simulink model "LQ_simulation"  (R2018a)
settings: Solver=ode45  StartTime=0.0  StopTime=50  RelTol=1e-3  EnableMultiTasking=on
values from neighbouring files (symbols this model uses):
  h = 0.001    [LQ_main.m]
  K = K_lqi(1:4)    [LQ_main.m]
  Ki = K_lqi(5:6)    [LQ_main.m]
  R_kal = cov(err)    [LQ_main.m]
undefined symbols (not defined in the file or in its folder): DiscIntNeverNeededParam, Discrete, get, hot, Time
libraries: simulink x2, ctrlSharedLib x1, dspmtrx3 x1, dspsnks4 x1
settings Model: Creator=rbabuska  LastModifiedBy=sstroobants
settings DataIOCC: LimitDataPoints=on  SaveFormat=Array  SignalLoggingName=sigsOut
settings OptimizationCC: BooleanDataType=off  ExpressionDepthLimit=2147483647  InitFltsAndDblsToZero=on  LifeSpan=inf
settings DebuggingCC: SaveWithParameterizedLinksMsg=none  SignalResolutionControl=TryResolveAllWithWarning  MultiTaskDSMMsg=warning  MultiTaskCondExecSysMsg=none  AllowSymbolicDim=off  StateNameClashWarn=warning  SFUnexpectedBacktrackingDiag=warning  SFNoUnconditionalDefaultTransitionDiag=warning  SFExecutionAtInitializationDiag=none
settings HardwareCC: ProdBitPerPointer=32  ProdBitPerSizeT=32  ProdBitPerPtrDiffT=32  ProdLargestAtomicFloat=None  ProdIntDivRoundTo=Undefined  ProdEndianess=Unspecified  ProdWordSize=32  ProdHWDeviceType=32-bit Generic  TargetUnknown=on
settings ModelReferenceCC: PropagateSignalLabelsOutOfModel=off
settings CodeAppCC: StateflowObjectComments=on
settings GRTTargetCC: TargetFcnLib=ansi_tfl_tmw.mat  TargetLangStandard=C89/C90 (ANSI)  GeneratePreprocessorConditionals=Disable all  CombineOutputUpdateFcns=off  GRTInterface=on
settings ConfigComp: CovMetricSettings=dw  CovHtmlReporting=on  CovSaveCumulativeToWorkspaceVar=on  CovSaveSingleToWorkspaceVar=on  CovExternalEMLEnable=off

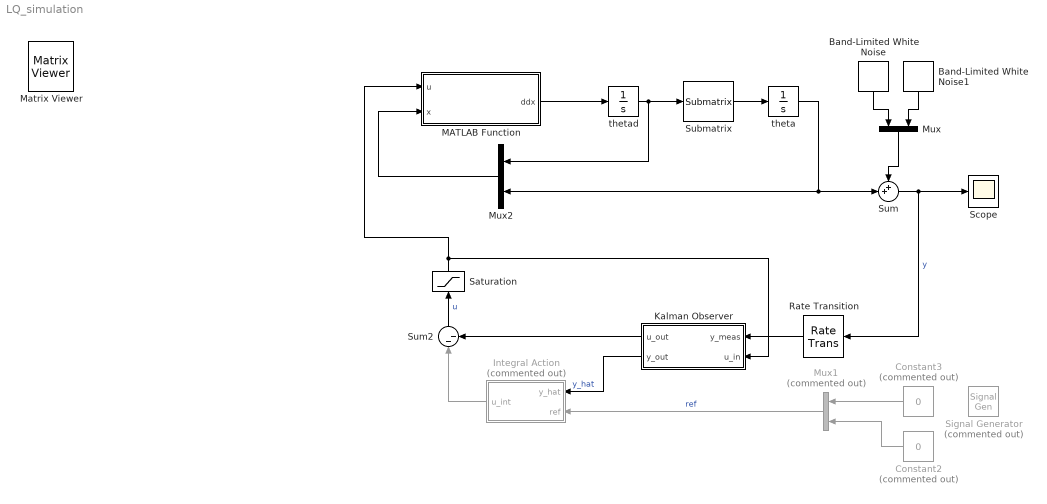
== system LQ_simulation ==
  Band-Limited White Noise : simulink/Sources/Band-Limited White Noise  Cov=R_kal(1,1)*h  Ts=h  seed=[23341]
  Band-Limited White Noise1 : simulink/Sources/Band-Limited White Noise  Cov=R_kal(2,2)*h  Ts=h  seed=[23341]
  Constant2 : Constant  Commented=on  Value=0
  Constant3 : Constant  Commented=on  Value=0
  Integral Action : Subsystem  Commented=on
  Kalman Observer : Subsystem
  MATLAB Function : MATLAB Function  TreatAsAtomicUnit=on  SystemSampleTime=h
  Mux : Mux  Inputs=2
  Mux1 : Mux  Commented=on  Inputs=2
  Mux2 : Mux  Inputs=2
  Rate Transition : RateTransition  OutPortSampleTime=h
  Saturation : Saturate  UpperLimit=1  LowerLimit=-1
  Scope : Scope
  Signal Generator : SignalGenerator  Commented=on  WaveForm=square  Amplitude=0.3  Frequency=0.2  Units=rad/sec
  Submatrix : dspmtrx3/Submatrix  RowSpan=Range of rows  RowStartMode=First  RowStartIndex=1  RowEndMode=Index  RowEndIndex=2  ColSpan=Range of columns  ColStartMode=First  ColStartIndex=1  ColEndMode=Last  ColEndIndex=1
  Sum : Sum  Inputs=++|
  Sum2 : Sum  Inputs=|--
  theta : Integrator  InitialCondition=[0;0]
  thetad : Integrator  InitialCondition=[0 0 0]
  Matrix Viewer : dspsnks4/Matrix Viewer  IOType=viewer  ImageParams=off  CMapStr=hot(256)  AxisColorbar=on  AxisParams=off  AxisOrigin=Upper left corner  AxisTickMode=Auto  XTickRange=[0 1]  YTickRange=[0 1]  XLabel=X-axis  YLabel=Y-axis  ZLabel=Z-axis  FigPos=get(0,'defaultfigureposition')  AxisZoom=off
      settings: SourceProductName=DSP System Toolbox  SourceProductBaseCode=DS  YMin=-1.0  YMax=1.0
  wires:
  Sum2/1 -> Saturation/1  "u"
  Saturation/1 -> MATLAB Function/1(u), Kalman Observer/2(u_in)
  Sum/1 -> Scope/1, Rate Transition/1  "y"
  Kalman Observer/1(u_out) -> Sum2/2
  Mux/1 -> Sum/1
  Band-Limited White Noise/1 -> Mux/1
  Band-Limited White Noise1/1 -> Mux/2
  Kalman Observer/2(y_out) -> Integral Action/1(y_hat)  "y_hat"
  Integral Action/1(u_int) -> Sum2/1
  Mux1/1 -> Integral Action/2(ref)  "ref"
  Constant2/1 -> Mux1/2
  Constant3/1 -> Mux1/1
  Mux2/1 -> MATLAB Function/2(x)
  Submatrix/1 -> theta/1
  thetad/1 -> Submatrix/1, Mux2/1
  MATLAB Function/1(ddx) -> thetad/1
  theta/1 -> Sum/2, Mux2/2
  Rate Transition/1 -> Kalman Observer/1(y_meas)

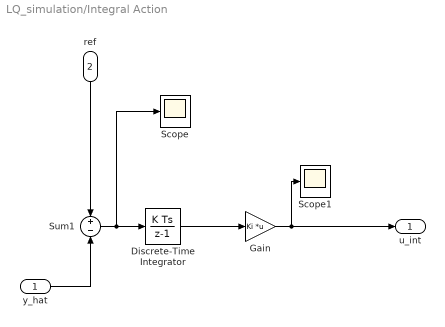
== system LQ_simulation/Integral Action ==
  y_hat : Inport
  ref : Inport  Port=2
  Discrete-Time Integrator : DiscreteIntegrator  gainval=1.5  SampleTime=h  ICPrevOutput=DiscIntNeverNeededParam  ICPrevScaledInput=DiscIntNeverNeededParam
  Gain : Gain  Gain=Ki  Multiplication=Matrix(K*u)
  Scope : Scope
  Scope1 : Scope
  Sum1 : Sum  Inputs=+-
  u_int : Outport
  wires:
  ref/1 -> Sum1/1
  y_hat/1 -> Sum1/2
  Sum1/1 -> Scope/1, Discrete-Time Integrator/1
  Discrete-Time Integrator/1 -> Gain/1
  Gain/1 -> Scope1/1, u_int/1

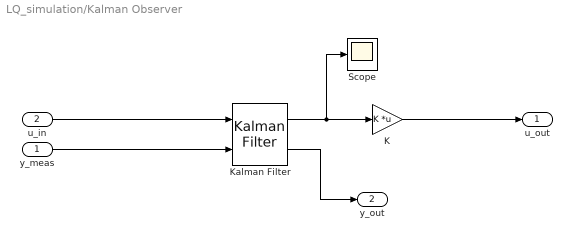
== system LQ_simulation/Kalman Observer ==
  y_meas : Inport  PortDimensions=2
  u_in : Inport  Port=2  PortDimensions=1  SampleTime=h
  K : Gain  Gain=K  Multiplication=Matrix(K*u)
  Kalman Filter : ctrlSharedLib/Kalman Filter  TimeDomain=Discrete-Time  UseCurrentEstimator=on  ModelSource=LTI State-Space Variable  ModelSourceVariable=sysd  A=0.95  B=1  C=1  D=0  NumberOfStates=1  NumberOfInputs=1  NumberOfOutputs=1  InitialEstimateSource=Dialog  X0=0  P0=10  UseK=off  UseGH=off  NumberOfProcessNoiseInputs=1  G=1  TimeInvariantG=on  H=0  TimeInvariantH=on  Q=10^(-7)*eye(4)  TimeInvariantQ=on  R=R_kal  TimeInvariantR=on  N=0  TimeInvariantN=on  AddInputPort=on  AddEnablePort=off  OutputEstimatedY=on  OutputP=off  Ts=-1
      settings: SourceProductBaseCode=CT
  Scope : Scope
  u_out : Outport
  y_out : Outport  Port=2
  wires:
  K/1 -> u_out/1
  u_in/1 -> Kalman Filter/1
  y_meas/1 -> Kalman Filter/2
  Kalman Filter/1 -> Scope/1, K/1
  Kalman Filter/2 -> y_out/1

== matlab function LQ_simulation/MATLAB Function ==
  data: u input; x input; ddx output
function ddx = nonlinsim(u,x)
theta1  = x(4);
theta2  = x(5);
theta1d = x(1);
theta2d = x(2);
ii      = x(3);
par =     [0.107001615392530   0.165343973632010   0.040783104942133   0.046364080778153   0.000051655820835   0.048856187724916   0.049137116812930   1.636038234993470   0.000031810472615   1.827977549139487   0.000008590269497   0.006045619229031   3.032790298604742   0.098524631245120   1.049678153165582];

%Define parameters
L1 = par(1);m1 = par(2);m2 = par(3); I1 = par(4); I2 = par(5);
c1 = par(6); c2 = par(7); 
b1 = par(8); b2 = par(9);  Bc1 = par(10); Bc2 = par(11);
 L = par(12); Kt = par(13); R = par(14); Kv = par(15);
g = 9.81;
M = -7;
%Input
Tau = u;%interp1(u.Time,u.Data,t);
ddx = zeros(3,1);
% dx(1) = x(3);
% dx(2) = x(4);
ddx(1) = (3*I2*Kt*ii - 2*Bc2*I2*atan(500*theta1d - 500*theta2d) - 2*Bc1*I2*atan(500*theta1d) - 3*I2*b1*theta1d - 3*I2*b2*theta1d + 3*I2*b2*theta2d - 2*Bc1*c2^2*m2*atan(500*theta1d) - 4*Bc2*c2^2*m2*atan(500*theta1d - 500*theta2d) + 3*Kt*c2^2*ii*m2 - 3*b1*c2^2*m2*theta1d - 6*b2*c2^2*m2*theta1d + 6*b2*c2^2*m2*theta2d + 3*L1*c2^2*g*m2^2*sin(theta1) + 3*I2*c2*g*m2*sin(theta1 + theta2) + 3*I2*L1*g*m2*sin(theta1) + 3*I2*c1*g*m1*sin(theta1) + 3*L1*c2^3*m2^2*theta1d^2*sin(theta2) + 3*L1*c2^3*m2^2*theta2d^2*sin(theta2) + 6*L1*c2^3*m2^2*theta1d*theta2d*sin(theta2) - 3*L1*b2*c2*m2*theta1d*cos(theta2) + 3*L1*b2*c2*m2*theta2d*cos(theta2) + 3*L1^2*c2^2*m2^2*theta1d^2*cos(theta2)*sin(theta2) - 3*L1*c2^2*g*m2^2*sin(theta1 + theta2)*cos(theta2) + 3*I2*L1*c2*m2*theta2d^2*sin(theta2) + 3*c1*c2^2*g*m1*m2*sin(theta1) - 2*Bc2*L1*c2*m2*atan(500*theta1d - 500*theta2d)*cos(theta2) + 6*I2*L1*c2*m2*theta1d*theta2d*sin(theta2))/(3*(I1*I2 + L1^2*c2^2*m2^2 + I2*L1^2*m2 + I1*c2^2*m2 + I2*c2^2*m2 - L1^2*c2^2*m2^2*cos(theta2)^2 + 2*I2*L1*c2*m2*cos(theta2)));
ddx(2) =  -(3*I1*b2*theta2d - 3*I1*b2*theta1d - 2*Bc2*I1*atan(500*theta1d - 500*theta2d) - 2*Bc1*c2^2*m2*atan(500*theta1d) - 2*Bc2*L1^2*m2*atan(500*theta1d - 500*theta2d) - 4*Bc2*c2^2*m2*atan(500*theta1d - 500*theta2d) + 3*Kt*c2^2*ii*m2 - 3*L1^2*b2*m2*theta1d + 3*L1^2*b2*m2*theta2d - 3*b1*c2^2*m2*theta1d - 6*b2*c2^2*m2*theta1d + 6*b2*c2^2*m2*theta2d - 3*L1^2*c2*g*m2^2*sin(theta1 + theta2) + 3*L1*c2^2*g*m2^2*sin(theta1) - 3*I1*c2*g*m2*sin(theta1 + theta2) + 3*L1*c2^3*m2^2*theta1d^2*sin(theta2) + 3*L1^3*c2*m2^2*theta1d^2*sin(theta2) + 3*L1*c2^3*m2^2*theta2d^2*sin(theta2) + 3*Kt*L1*c2*ii*m2*cos(theta2) + 6*L1*c2^3*m2^2*theta1d*theta2d*sin(theta2) - 3*L1*b1*c2*m2*theta1d*cos(theta2) - 9*L1*b2*c2*m2*theta1d*cos(theta2) + 9*L1*b2*c2*m2*theta2d*cos(theta2) + 6*L1^2*c2^2*m2^2*theta1d^2*cos(theta2)*sin(theta2) + 3*L1^2*c2^2*m2^2*theta2d^2*cos(theta2)*sin(theta2) - 3*L1*c2^2*g*m2^2*sin(theta1 + theta2)*cos(theta2) + 3*L1^2*c2*g*m2^2*cos(theta2)*sin(theta1) + 3*I1*L1*c2*m2*theta1d^2*sin(theta2) + 3*c1*c2^2*g*m1*m2*sin(theta1) - 2*Bc1*L1*c2*m2*atan(500*theta1d)*cos(theta2) - 6*Bc2*L1*c2*m2*atan(500*theta1d - 500*theta2d)*cos(theta2) + 6*L1^2*c2^2*m2^2*theta1d*theta2d*cos(theta2)*sin(theta2) + 3*L1*c1*c2*g*m1*m2*cos(theta2)*sin(theta1))/(3*(I1*I2 + L1^2*c2^2*m2^2 + I2*L1^2*m2 + I1*c2^2*m2 + I2*c2^2*m2 - L1^2*c2^2*m2^2*cos(theta2)^2 + 2*I2*L1*c2*m2*cos(theta2)));
ddx(3) = -(R*ii - M*Tau + Kv*theta1d)/L;
% dx = dx';

end
